simulink model "obstacle_holding_file"  (Simulink 7.5)
settings: Solver=ode45  StartTime=0.0  StopTime=10.0  RelTol=1e-3
undefined symbols (not defined in the file or in its folder): CR, serial
libraries: instrumentlib x2
settings Model: Creator=bujiie  LastModifiedBy=bujiie

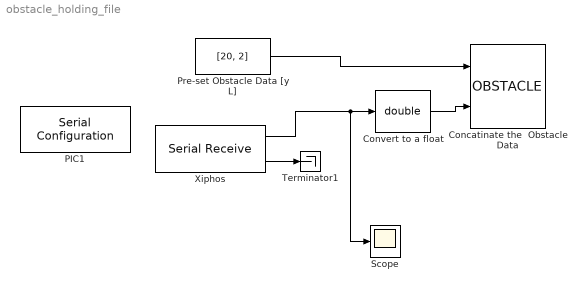
== system obstacle_holding_file ==
  Concatinate the  Obstacle Data : M-S-Function  FunctionName=OBSTACLE  Parameters=2
  Convert to a float : DataTypeConversion  OutDataTypeMode=double  OutDataTypeStr=double  SaturateOnIntegerOverflow=on  RndMeth=Zero
  PIC1 : instrumentlib/Serial Configuration  Priority=-200000  DialogController=instrumentcreatedialog  DialogControllerArgs=DataTag0  ComPortMenu=<Please select a port...>  ComPort=COM5  ObjConstructor=serial('COM5');  BaudRate=9600  DataBits=8  Parity=none  StopBits=1  FlowControl=none  Timeout=10  ByteOrder=LittleEndian
  Pre-set Obstacle Data [y L] : Constant  Value=[20, 2]  OutDataType=fixdt(1, 16)  OutScaling=2^0  SampleTime=.05
  Scope : Scope
      settings: YMin=-1  YMax=1
  Terminator1 : Terminator
  Xiphos : instrumentlib/Serial Receive  DialogController=instrumentcreatedialog  DialogControllerArgs=DataTag1  ComPortMenu=<Please select a port...>  ComPort=COM5  ObjConstructor=serial('COM5');  Terminator=CR ('\r')  DataSize="[1  3]"  DataType=int8  EnableBlockingMode=off  ActionDataUnavailable=Output last received value  CustomValue=0  SampleTime=0.05
  wires:
  Pre-set Obstacle Data [y L]/1 -> Concatinate the  Obstacle Data/1
  Convert to a float/1 -> Concatinate the  Obstacle Data/2
  Xiphos/2 -> Terminator1/1
  Xiphos/1 -> Convert to a float/1, Scope/1
